simulink model "Pure_Pursuit_With_VFH"  (R2017b)
settings: Solver=FixedStepAuto  StartTime=0.0  StopTime=10.0  FixedStep=0.05  RelTol=1e-3
model workspace (MAT data in the model file):
  SL_ROS_VariableLengthArrays_MaxSizes.CommonInfo.ArrayTruncateAction = 'EmitWarning'
  SL_ROS_VariableLengthArrays_MaxSizes.MsgTypeMap = containers.Map
  SL_ROS_VariableLengthArrays_MaxSizes.MsgTypeMap.serialization.keys = {'sensor_msgs/LaserScan', 'std_msgs/Header'}
  SL_ROS_VariableLengthArrays_MaxSizes.MsgTypeMap.serialization.values{1}(1).PropertyName = 'Intensities'
  SL_ROS_VariableLengthArrays_MaxSizes.MsgTypeMap.serialization.values{1}(1).DataType = 'single'
  SL_ROS_VariableLengthArrays_MaxSizes.MsgTypeMap.serialization.values{1}(1).MaxLength = 721
  SL_ROS_VariableLengthArrays_MaxSizes.MsgTypeMap.serialization.values{1}(2).PropertyName = 'Ranges'
  SL_ROS_VariableLengthArrays_MaxSizes.MsgTypeMap.serialization.values{1}(2).DataType = 'single'
  SL_ROS_VariableLengthArrays_MaxSizes.MsgTypeMap.serialization.values{1}(2).MaxLength = 721
  SL_ROS_VariableLengthArrays_MaxSizes.MsgTypeMap.serialization.values{2}.PropertyName = 'FrameId'
  SL_ROS_VariableLengthArrays_MaxSizes.MsgTypeMap.serialization.values{2}.DataType = 'uint8'
  SL_ROS_VariableLengthArrays_MaxSizes.MsgTypeMap.serialization.values{2}.MaxLength = 720
  SL_ROS_VariableLengthArrays_MaxSizes.MsgTypeMap.serialization.uniformity = 0
  SL_ROS_VariableLengthArrays_MaxSizes.MsgTypeMap.serialization.keyType = 'char'
  SL_ROS_VariableLengthArrays_MaxSizes.MsgTypeMap.serialization.valueType = 'any'
  lookahead_dist = Simulink.Parameter
  lookahead_dist.Value = 2
  lookahead_dist.DataType = 'auto'
  lookahead_dist.Dimensions = [1 1]
undefined symbols (not defined in the file): Angular, Linear
libraries: robotlib x7, simulink x5, robotalgslib x2, simulink_extras x1, dspsigops x1
settings Model: ExplicitPartitioning=on  Creator=andrej  LastModifiedBy=andrej
settings OptimizationCC: PassReuseOutputArgsThreshold=0  MaxStackSize=64
settings DebuggingCC: ParameterTunabilityLossMsg=error
settings HardwareCC: ProdBitPerLong=64  ProdHWDeviceType=Intel->x86-64 (Linux 64)  UseEmbeddedCoderFeatures=off
settings SFSimCC: MATLABDynamicMemAlloc=off
settings RTWCC: SystemTargetFile=ert.tlc  HardwareBoard=Robot Operating System (ROS)  TemplateMakefile=ert_default_tmf  GenerateReport=on  Toolchain=Catkin  BuildConfiguration=Faster Runs  LaunchReport=on  TargetLang=C++
settings RTWCC: CustomInitializer=|
  | ros::NodeHandle private_nh = ros::NodeHandle("~");
  | 	ROS_INFO_STREAM("Node's namespace: " << private_nh.getNamespace());
  | 
  | // Tunable parameters of the Pure Pursuit algorithm
  | 	double desired_lin_vel;
  | 	if (private_nh.getParam("pure_pursuit/desired_lin_vel", desired_lin_vel))
  | 		this->Pure_Pursuit_With_VFH_P.PurePursuit_DesiredLinearVeloci = desired_lin_vel;
  | 	ROS_WARN_STREAM("Pure pursuit desired linear velocity set to " << this->Pure_Pursuit_With_VFH_P.PurePursuit_DesiredLinearVeloci << " m/s.");
  | 	double max_ang_vel;
  | 	if (private_nh.getParam("pure_pursuit/max_ang_vel", max_ang_vel))
  | 		this->Pure_Pursuit_With_VFH_P.PurePursuit_MaxAngularVelocity = max_ang_vel;
  | 	this->Pure_Pursuit_With_VFH_P.MaxAngularVelocity_Value = this->Pure_Pursuit_With_VFH_P.PurePursuit_MaxAngularVelocity;
  | 	double lookahead_dist;
  | 	if (private_nh.getParam("pure_pursuit/lookahead_dist", lookahead_dist))
  | 		this->Pure_Pursuit_With_VFH_P.PurePursuit_LookaheadDistance = lookahead_dist;
  | 
  | // Goal reach tolerance
  | 	double goal_radius;
  | 	if (private_nh.getParam("goal_radius", goal_radius))
  | 		this->Pure_Pursuit_With_VFH_P.GoalRadius_Value = goal_radius;
  | 
  | 
  | // Tunable parameters of the VFH algorithm
  | 
  | 	std::vector<double> range_dist;
  | 	if (private_nh.getParam("vfh/range_dist", range_dist)) {
  | 		this->Pure_Pursuit_With_VFH_P.VectorFieldHistogram_DistanceLi[0] = range_dist[0];
  | 		this->Pure_Pursuit_With_VFH_P.VectorFieldHistogram_DistanceLi[1] = range_dist[1];
  | 	}
  | 	std::vector<double> hist_thr;
  | 	if (private_nh.getParam("vfh/hist_thr", hist_thr)) {
  | 		this->Pure_Pursuit_With_VFH_P.VectorFieldHistogram_HistogramT[0] = hist_thr[0];
  | 		this->Pure_Pursuit_With_VFH_P.VectorFieldHistogram_HistogramT[1] = hist_thr[1];
  | 	}
  | 	double robot_radius;
  | 	if (private_nh.getParam("vfh/robot_radius", robot_radius))
  | 		this->Pure_Pursuit_With_VFH_P.VectorFieldHistogram_RobotRadiu = robot_radius;
  | 	double safety_dist;
  | 	if (private_nh.getParam("vfh/safety_dist", safety_dist))
  | 		this->Pure_Pursuit_With_VFH_P.VectorFieldHistogram_SafetyDist = safety_dist;
  | 	double min_turning_radius;
  | 	if (private_nh.getParam("vfh/min_turning_radius", min_turning_radius))
  | 		this->Pure_Pursuit_With_VFH_P.VectorFieldHistogram_MinTurning = min_turning_radius;
  | 	double target_dir_w;
  | 	if (private_nh.getParam("vfh/target_dir_w", target_dir_w))
  | 		this->Pure_Pursuit_With_VFH_P.VectorFieldHistogram_TargetDire = target_dir_w;
  | 	double current_dir_w;
  | 	if (private_nh.getParam("vfh/current_dir_w", current_dir_w))
  | 		this->Pure_Pursuit_With_VFH_P.VectorFieldHistogram_CurrentDir = current_dir_w;
  | 	double prev_dir_w;
  | 	if (private_nh.getParam("vfh/prev_dir_w", prev_dir_w))
  | 		this->Pure_Pursuit_With_VFH_P.VectorFieldHistogram_PreviousDi = prev_dir_w;
  | 
  | // Tunable parameters of the Linear Velocity Control
  | double double_param;
  | bool bool_param;
  | 
  | 	if (private_nh.getParam("velocity_profile/a", double_param))
  | 		this->Pure_Pursuit_With_VFH_P.LinVelocityControl_a = double_param;
  | 
  | 	if (private_nh.getParam("velocity_profile/c", double_param))
  | 		this->Pure_Pursuit_With_VFH_P.LinVelocityControl_c = double_param;
  | 
  |         if (private_nh.getParam("velocity_profile/k", double_param))
  | 		this->Pure_Pursuit_With_VFH_P.LinVelocityControl_k = double_param;
  | 
  | 	this->Pure_Pursuit_With_VFH_P.LinVelocityControl_omega_max = this->Pure_Pursuit_With_VFH_P.PurePursuit_MaxAngularVelocity;
  | 
  | 	if (private_nh.getParam("velocity_profile/v_max", double_param))
  | 		this->Pure_Pursuit_With_VFH_P.LinVelocityControl_v_max = double_param;
  | 
  | 	if (private_nh.getParam("velocity_profile/v_min", double_param))
  | 		this->Pure_Pursuit_With_VFH_P.LinVelocityControl_v_min = double_param;
  | 
  | 	if (private_nh.getParam("velocity_profile/enable", bool_param))
  | 		this->Pure_Pursuit_With_VFH_P.LinVelocityControl_enable = bool_param;
settings CodeAppCC: ForceParamTrailComments=on  OperatorAnnotations=on  StateflowObjectComments=on
settings ERTTargetCC: CodeReplacementLibrary=Intel IPP for x86-64 (Linux)  ERTCustomFileBanners=off  MultiInstanceERTCode=on  CodeInterfacePackaging=C++ class  SupportContinuousTime=on  SupportNonInlinedSFcns=on  RemoveResetFunc=off  ModelStepFunctionPrototypeControlCompliant=off  IndentSize=4

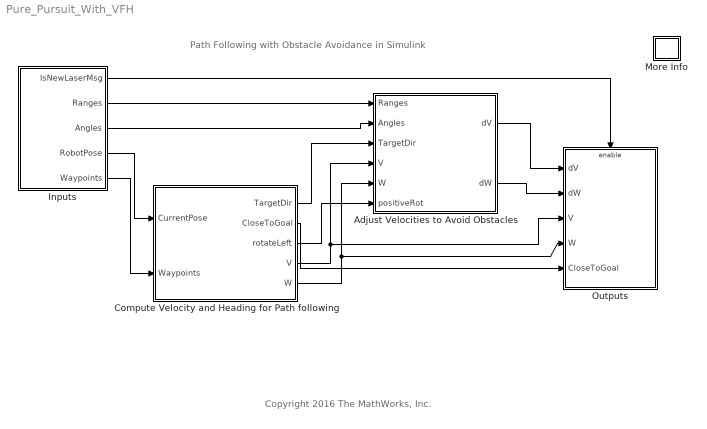
== system Pure_Pursuit_With_VFH ==
  note: Copyright 2016 The MathWorks, Inc.
  note: Path Following with Obstacle Avoidance in Simulink
  Adjust Velocities to Avoid Obstacles : Subsystem
  Compute Velocity and Heading for Path following : Subsystem
  Inputs : Subsystem
  More Info : Subsystem
      settings: OpenFcn=showdemo(bdroot(gcb))
      mask Display: disp('?')
  Outputs : Subsystem
  wires:
  Compute Velocity and Heading for Path following/2(CloseToGoal) -> Outputs/5(CloseToGoal)
  Inputs/5(Waypoints) -> Compute Velocity and Heading for Path following/2(Waypoints)
  Inputs/4(RobotPose) -> Compute Velocity and Heading for Path following/1(CurrentPose)
  Inputs/1(IsNewLaserMsg) -> Outputs/Enable
  Inputs/2(Ranges) -> Adjust Velocities to Avoid Obstacles/1(Ranges)
  Adjust Velocities to Avoid Obstacles/2(dW) -> Outputs/2(dW)
  Compute Velocity and Heading for Path following/1(TargetDir) -> Adjust Velocities to Avoid Obstacles/3(TargetDir)
  Inputs/3(Angles) -> Adjust Velocities to Avoid Obstacles/2(Angles)
  Compute Velocity and Heading for Path following/3(rotateLeft) -> Adjust Velocities to Avoid Obstacles/6(positiveRot)
  Adjust Velocities to Avoid Obstacles/1(dV) -> Outputs/1(dV)
  Compute Velocity and Heading for Path following/5(W) -> Adjust Velocities to Avoid Obstacles/5(W), Outputs/4(W)
  Compute Velocity and Heading for Path following/4(V) -> Adjust Velocities to Avoid Obstacles/4(V), Outputs/3(V)

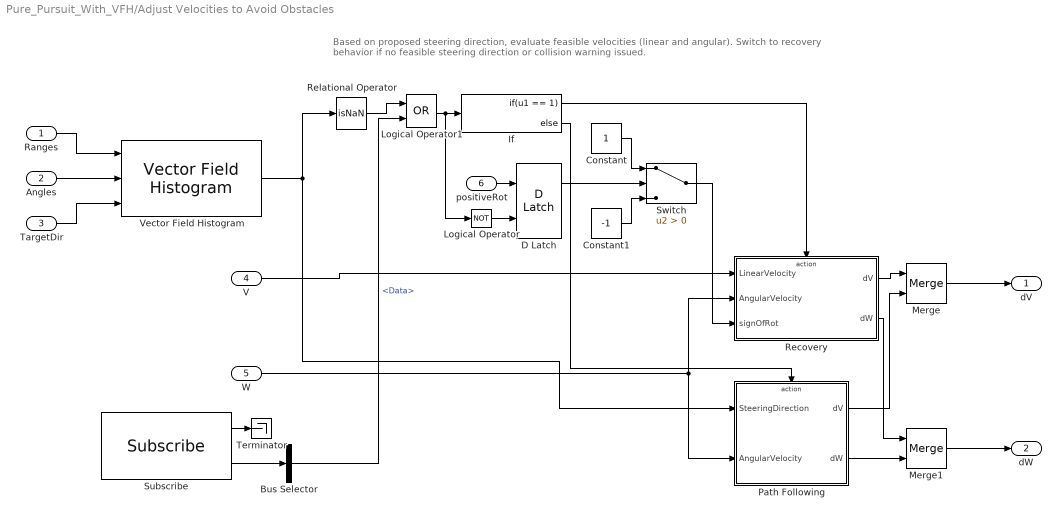
== system Pure_Pursuit_With_VFH/Adjust Velocities to Avoid Obstacles ==
  note: Based on proposed steering direction, evaluate feasible velocities (linear and angular).
      | 	Switch to recovery behavior if no feasible steering direction or collision warning issued.
  Ranges : Inport
  Angles : Inport  Port=2
  TargetDir : Inport  Port=3
  V : Inport  Port=4
  W : Inport  Port=5
  positiveRot : Inport  Port=6
  Bus Selector : BusSelector  OutputSignals=Data
  Constant : Constant
  Constant1 : Constant  Value=-1
  D Latch : simulink_extras/Flip Flops/D Latch
      settings: SourceProductName=Simulink  SourceProductBaseCode=SL
  If : If  IfExpression=u1 == 1
  Logical Operator : Logic  Operator=NOT  IconShape=distinctive  AllPortsSameDT=off  OutDataTypeStr=boolean
  Logical Operator1 : Logic  Operator=OR  AllPortsSameDT=off  OutDataTypeStr=boolean
  Merge : Merge
  Merge1 : Merge
  Path Following : Subsystem  TreatAsAtomicUnit=on
  Recovery : Subsystem  TreatAsAtomicUnit=on
  Relational Operator : RelationalOperator  Operator=isNaN  OutDataTypeStr=boolean  RndMeth=Simplest
  Subscribe : robotlib/Subscribe  SourceLibraryInfo=This block requires Robotics System Toolbox  topicSource=Specify your own  topic=/Collision_warning  messageType=std_msgs/Bool  sampleTime=-1  messageQueueLength=1
      settings: SourceProductBaseCode=RO
  Switch : Switch  Criteria=u2 > Threshold
  Terminator : Terminator
  Vector Field Histogram : robotalgslib/Vector Field Histogram  NumAngularSectors=240  DistanceLimits=[ 0.05, 2.0 ]  HistogramThresholds=[ 3, 6 ]  RobotRadius=0.3  SafetyDistance=0.1  MinTurningRadius=0.3  SimulateUsing=Code generation  TargetDirectionWeight=5  CurrentDirectionWeight=2  PreviousDirectionWeight=2
      settings: SourceProductName=Robotics System Toolbox  SourceProductBaseCode=RO
  dV : Outport
  dW : Outport  Port=2
  wires:
  Merge1/1 -> dW/1
  V/1 -> Recovery/1(LinearVelocity)
  Vector Field Histogram/1 -> Path Following/1(SteeringDirection), Relational Operator/1
  W/1 -> Path Following/2(AngularVelocity), Recovery/2(AngularVelocity)
  Angles/1 -> Vector Field Histogram/2
  Merge/1 -> dV/1
  TargetDir/1 -> Vector Field Histogram/3
  Ranges/1 -> Vector Field Histogram/1
  If/1 -> Recovery/Action
  If/2 -> Path Following/Action
  Recovery/2(dW) -> Merge1/1
  Path Following/2(dW) -> Merge1/2
  Recovery/1(dV) -> Merge/1
  Path Following/1(dV) -> Merge/2
  Subscribe/2 -> Bus Selector/1
  Subscribe/1 -> Terminator/1
  Logical Operator1/1 -> Logical Operator/1, If/1
  Relational Operator/1 -> Logical Operator1/1
  Bus Selector/1 -> Logical Operator1/2  "<Data>"
  Logical Operator/1 -> D Latch/2
  positiveRot/1 -> D Latch/1
  D Latch/1 -> Switch/2
  Switch/1 -> Recovery/3(signOfRot)
  Constant/1 -> Switch/1
  Constant1/1 -> Switch/3

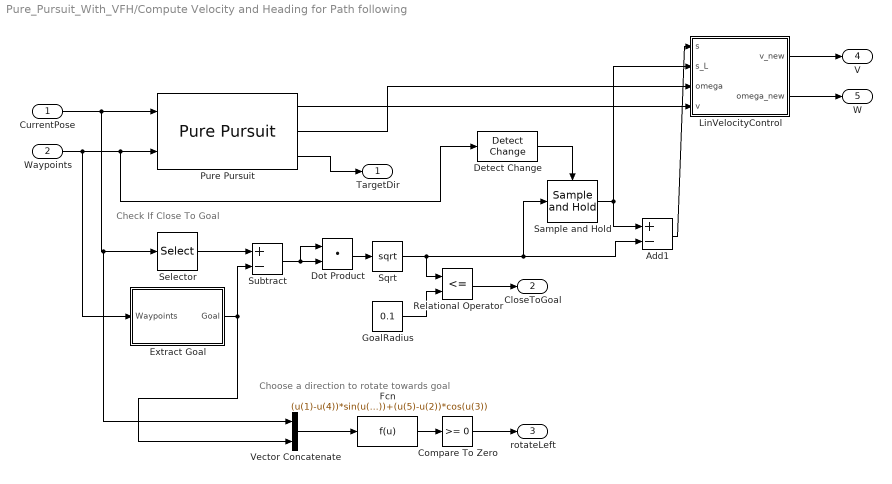
== system Pure_Pursuit_With_VFH/Compute Velocity and Heading for Path following ==
  note: Choose a direction to rotate towards goal
  note: Check If Close To Goal
  CurrentPose : Inport
  Waypoints : Inport  Port=2
  " Extract Goal" : MATLAB Function  TreatAsAtomicUnit=on
  Add1 : Sum  Inputs=+-
  Compare To Zero : simulink/Logic and Bit Operations/Compare To Zero  relop=>=  OutDataTypeStr=boolean
  Detect Change : simulink/Logic and Bit Operations/Detect Change  vinit=true  OutDataTypeStr=boolean
  Dot Product : DotProduct  InputSameDT=on  OutDataTypeStr=Inherit: Inherit via internal rule
  Fcn : Fcn  Expr=(u(1)-u(4))*sin(u(3))+(u(5)-u(2))*cos(u(3))
  GoalRadius : Constant  Value=0.1
  LinVelocityControl : Subsystem  mask(Desired velocity profile){v_min=0.2, v_max=0.9, omega_max=1.0, c=0.5, a=0.3, k=10, enable=on}
      mask prompts: v_min "v_min [m/s]"; v_max "v_max [m/s]"; omega_max "omega_max [rad/s]"; c "c [m]"; a "a [m/s^2]"; k "Prefilter constant k"; enable "enable control"
      mask help:
      | Robot moves with velocity v_min around the waypoints (+/- c) and accelerating with constant acceleration (a) in between.
      | Maximum speed is  v_max.
      | Reference prefilter has the transfer function of the form k/(s+k).
      | Enable control to change velocity according to this profile, otherwise pass through velocity inputs.
  Pure Pursuit : robotalgslib/Pure Pursuit  DesiredLinearVelocity=0.3  MaxAngularVelocity=1.0  LookaheadDistance=1.0  TargetDirPort=on  SimulateUsing=Code generation
      settings: SourceProductName=Robotics System Toolbox  SourceProductBaseCode=RO
  Relational Operator : RelationalOperator  Operator=<=  OutDataTypeStr=boolean  RndMeth=Simplest
  Sample and Hold : dspsigops/Sample and Hold  trig=Rising edge  initCond=0  latchinput=off
  Selector : Selector  InputPortWidth=3  IndexOptions=Index vector (dialog)  Indices=[1 2]  OutputSizes=1
  Sqrt : Sqrt  SaturateOnIntegerOverflow=on
  Subtract : Sum  Inputs=+-
  Vector Concatenate : Concatenate
  TargetDir : Outport
  CloseToGoal : Outport  Port=2
  rotateLeft : Outport  Port=3
  V : Outport  Port=4
  W : Outport  Port=5
  wires:
  Pure Pursuit/3 -> TargetDir/1
  Waypoints/1 -> " Extract Goal"/1(Waypoints), Detect Change/1, Pure Pursuit/2
  CurrentPose/1 -> Vector Concatenate/1, Selector/1, Pure Pursuit/1
  Relational Operator/1 -> CloseToGoal/1
  GoalRadius/1 -> Relational Operator/2
  Selector/1 -> Subtract/1
  Dot Product/1 -> Sqrt/1
  Sqrt/1 -> Sample and Hold/1, Add1/2, Relational Operator/1
  Subtract/1 -> Dot Product/1, Dot Product/2
  " Extract Goal"/1(Goal) -> Subtract/2, Vector Concatenate/2
  Vector Concatenate/1 -> Fcn/1
  Fcn/1 -> Compare To Zero/1
  Compare To Zero/1 -> rotateLeft/1
  Detect Change/1 -> Sample and Hold/Trigger
  Sample and Hold/1 -> Add1/1, LinVelocityControl/2(s_L)
  Add1/1 -> LinVelocityControl/1(s)
  LinVelocityControl/1(v_new) -> V/1
  LinVelocityControl/2(omega_new) -> W/1
  Pure Pursuit/2 -> LinVelocityControl/3(omega)
  Pure Pursuit/1 -> LinVelocityControl/4(v)

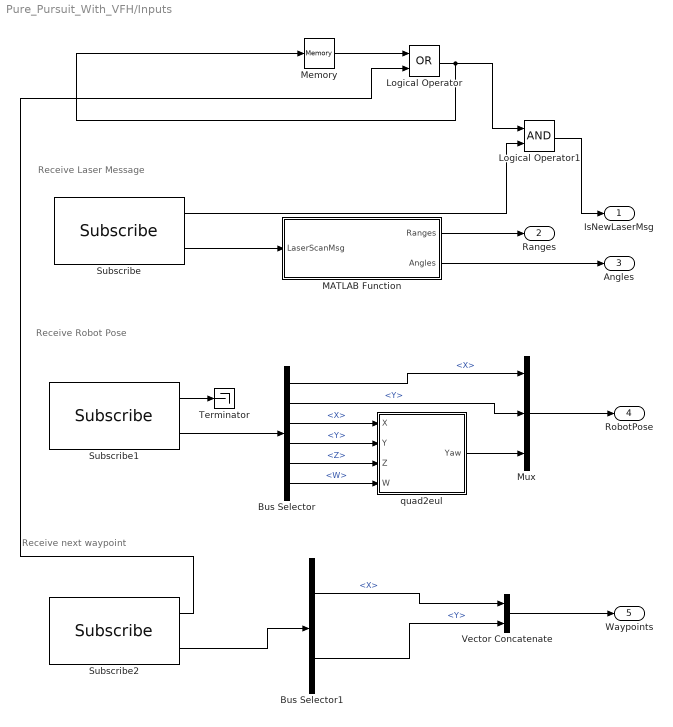
== system Pure_Pursuit_With_VFH/Inputs ==
  note: Receive next waypoint
  note: Receive Robot Pose
  note: Receive Laser Message
  Bus Selector : BusSelector  OutputSignals=Pose.Pose.Position.X,Pose.Pose.Position.Y,Pose.Pose.Orientation.X,Pose.Pose.Orientation.Y,Pose.Pose.Orientation.Z,Pose.Pose.Orientation.W
  Bus Selector1 : BusSelector  OutputSignals=X,Y
  Logical Operator : Logic  Operator=OR  AllPortsSameDT=off  OutDataTypeStr=boolean
  Logical Operator1 : Logic  AllPortsSameDT=off  OutDataTypeStr=boolean
  MATLAB Function : MATLAB Function  TreatAsAtomicUnit=on
  Memory : Memory
  Mux : Mux  Inputs=3
  Subscribe : robotlib/Subscribe  SourceLibraryInfo=This block requires Robotics System Toolbox  topicSource=Select from ROS network  topic=/scan  messageType=sensor_msgs/LaserScan  sampleTime=-1  messageQueueLength=1
      settings: SourceProductBaseCode=RO
  Subscribe1 : robotlib/Subscribe  SourceLibraryInfo=This block requires Robotics System Toolbox  topicSource=Specify your own  topic=/current_pose  messageType=nav_msgs/Odometry  sampleTime=-1  messageQueueLength=1
      settings: SourceProductBaseCode=RO
  Subscribe2 : robotlib/Subscribe  SourceLibraryInfo=This block requires Robotics System Toolbox  topicSource=Specify your own  topic=/next_waypoint  messageType=geometry_msgs/Point  sampleTime=-1  messageQueueLength=1
      settings: SourceProductBaseCode=RO
  Terminator : Terminator
  Vector Concatenate : Concatenate  Mode=Multidimensional array  ConcatenateDimension=2
  quad2eul : MATLAB Function  TreatAsAtomicUnit=on
  IsNewLaserMsg : Outport
  Ranges : Outport  Port=2
  Angles : Outport  Port=3
  RobotPose : Outport  Port=4
  Waypoints : Outport  Port=5
  wires:
  Subscribe/2 -> MATLAB Function/1(LaserScanMsg)
  quad2eul/1(Yaw) -> Mux/3
  Subscribe1/2 -> Bus Selector/1
  Bus Selector/3 -> quad2eul/1(X)  "<X>"
  Subscribe1/1 -> Terminator/1
  Bus Selector/2 -> Mux/2  "<Y>"
  Bus Selector/5 -> quad2eul/3(Z)  "<Z>"
  Bus Selector/4 -> quad2eul/2(Y)  "<Y>"
  Bus Selector/1 -> Mux/1  "<X>"
  Bus Selector/6 -> quad2eul/4(W)  "<W>"
  MATLAB Function/1(Ranges) -> Ranges/1
  MATLAB Function/2(Angles) -> Angles/1
  Subscribe/1 -> Logical Operator1/2
  Mux/1 -> RobotPose/1
  Subscribe2/2 -> Bus Selector1/1
  Bus Selector1/1 -> Vector Concatenate/1  "<X>"
  Bus Selector1/2 -> Vector Concatenate/2  "<Y>"
  Vector Concatenate/1 -> Waypoints/1
  Memory/1 -> Logical Operator/1
  Logical Operator/1 -> Logical Operator1/1, Memory/1
  Subscribe2/1 -> Logical Operator/2
  Logical Operator1/1 -> IsNewLaserMsg/1

== system Pure_Pursuit_With_VFH/More Info ==

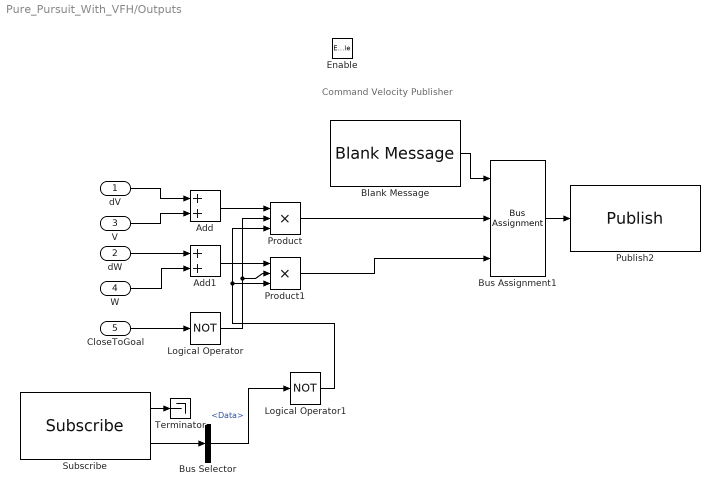
== system Pure_Pursuit_With_VFH/Outputs ==
  note: Command Velocity Publisher
  dV : Inport
  dW : Inport  Port=2
  V : Inport  Port=3
  W : Inport  Port=4
  CloseToGoal : Inport  Port=5
  Enable : EnablePort
  Add : Sum
  Add1 : Sum
  Blank Message : robotlib/Blank Message  SourceLibraryInfo=This block requires Robotics System Toolbox  messageType=geometry_msgs/Twist  SampleTime=inf
      settings: SourceProductBaseCode=RO
  Bus Assignment1 : BusAssignment  DialogController=Simulink.DDGSource_BusAssignment  AssignedSignals=Linear.X,Angular.Z
  Bus Selector : BusSelector  OutputSignals=Data
  Logical Operator : Logic  Operator=NOT  AllPortsSameDT=off  OutDataTypeStr=boolean
  Logical Operator1 : Logic  Operator=NOT  AllPortsSameDT=off  OutDataTypeStr=boolean
  Product : Product  Inputs=3
  Product1 : Product  Inputs=3
  Publish2 : robotlib/Publish  SourceLibraryInfo=This block requires Robotics System Toolbox  topicSource=Select from ROS network  topic=/mobile_base/commands/velocity  messageType=geometry_msgs/Twist  messageQueueLength=1
      settings: SourceProductBaseCode=RO
  Subscribe : robotlib/Subscribe  SourceLibraryInfo=This block requires Robotics System Toolbox  topicSource=Specify your own  topic=/emergency_stop  messageType=std_msgs/Bool  sampleTime=-1  messageQueueLength=1
      settings: SourceProductBaseCode=RO
  Terminator : Terminator
  wires:
  V/1 -> Add/2
  W/1 -> Add1/2
  dV/1 -> Add/1
  dW/1 -> Add1/1
  CloseToGoal/1 -> Logical Operator/1
  Add/1 -> Product/1
  Add1/1 -> Product1/1
  Product1/1 -> Bus Assignment1/3
  Product/1 -> Bus Assignment1/2
  Blank Message/1 -> Bus Assignment1/1
  Bus Assignment1/1 -> Publish2/1
  Logical Operator/1 -> Product1/2, Product/2
  Logical Operator1/1 -> Product1/3, Product/3
  Subscribe/2 -> Bus Selector/1
  Bus Selector/1 -> Logical Operator1/1  "<Data>"
  Subscribe/1 -> Terminator/1

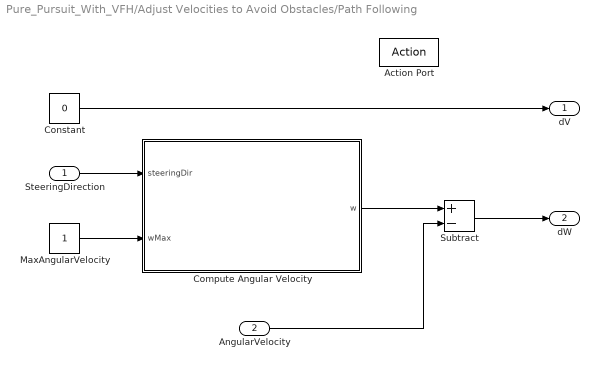
== system Pure_Pursuit_With_VFH/Adjust Velocities to Avoid Obstacles/Path Following ==
  SteeringDirection : Inport
  AngularVelocity : Inport  Port=2
  Action Port : ActionPort  ActionType=else
  Compute Angular Velocity : MATLAB Function  TreatAsAtomicUnit=on
  Constant : Constant  Value=0
  MaxAngularVelocity : Constant
  Subtract : Sum  Inputs=+-
  dV : Outport
  dW : Outport  Port=2
  wires:
  Constant/1 -> dV/1
  MaxAngularVelocity/1 -> Compute Angular Velocity/2(wMax)
  SteeringDirection/1 -> Compute Angular Velocity/1(steeringDir)
  Subtract/1 -> dW/1
  Compute Angular Velocity/1(w) -> Subtract/1
  AngularVelocity/1 -> Subtract/2

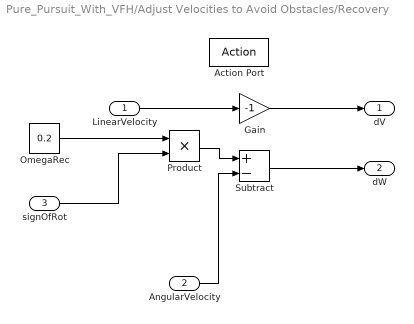
== system Pure_Pursuit_With_VFH/Adjust Velocities to Avoid Obstacles/Recovery ==
  LinearVelocity : Inport
  AngularVelocity : Inport  Port=2
  signOfRot : Inport  Port=3
  Action Port : ActionPort  ActionType=then
  Gain : Gain  Gain=-1
  OmegaRec : Constant  Value=0.2
  Product : Product
  Subtract : Sum  Inputs=+-
  dV : Outport
  dW : Outport  Port=2
  wires:
  LinearVelocity/1 -> Gain/1
  Gain/1 -> dV/1
  Subtract/1 -> dW/1
  OmegaRec/1 -> Product/1
  Product/1 -> Subtract/1
  AngularVelocity/1 -> Subtract/2
  signOfRot/1 -> Product/2

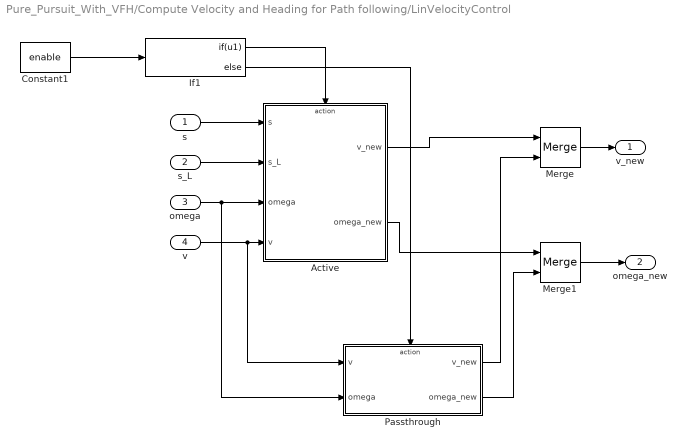
== system Pure_Pursuit_With_VFH/Compute Velocity and Heading for Path following/LinVelocityControl ==
  s : Inport
  s_L : Inport  Port=2
  omega : Inport  Port=3
  v : Inport  Port=4
  Active : Subsystem  TreatAsAtomicUnit=on
      mask Display: image('Vel_Profile.svg');
  Constant1 : Constant  Value=enable  OutDataTypeStr=boolean
  If1 : If  IfExpression=u1
  Merge : Merge
  Merge1 : Merge
  Passthrough : Subsystem  TreatAsAtomicUnit=on
  v_new : Outport
  omega_new : Outport  Port=2
  wires:
  s/1 -> Active/1(s)
  s_L/1 -> Active/2(s_L)
  omega/1 -> Passthrough/2(omega), Active/3(omega)
  v/1 -> Passthrough/1(v), Active/4(v)
  Constant1/1 -> If1/1
  If1/1 -> Active/Action
  If1/2 -> Passthrough/Action
  Merge/1 -> v_new/1
  Active/1(v_new) -> Merge/1
  Passthrough/1(v_new) -> Merge/2
  Active/2(omega_new) -> Merge1/1
  Passthrough/2(omega_new) -> Merge1/2
  Merge1/1 -> omega_new/1

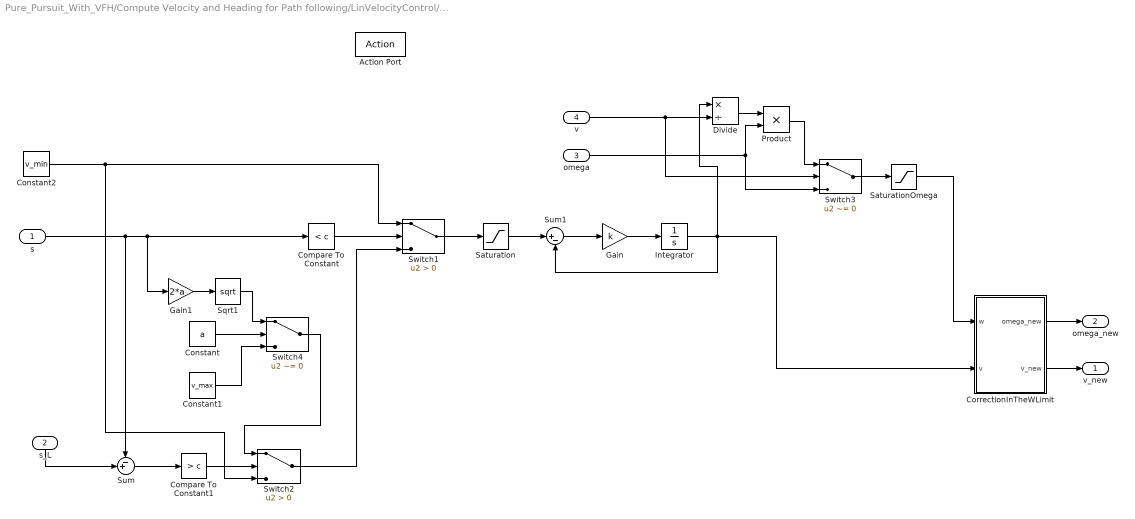
== system Pure_Pursuit_With_VFH/Compute Velocity and Heading for Path following/LinVelocityControl/Active ==
  s : Inport
  s_L : Inport  Port=2
  omega : Inport  Port=3
  v : Inport  Port=4
  Action Port : ActionPort  ActionType=then
  Compare To Constant : simulink/Logic and Bit Operations/Compare To Constant  relop=<  const=c  OutDataTypeStr=boolean
  Compare To Constant1 : simulink/Logic and Bit Operations/Compare To Constant  relop=>  const=c  OutDataTypeStr=boolean
  Constant : Constant  Value=a
  Constant1 : Constant  Value=v_max
  Constant2 : Constant  Value=v_min
  CorrectionInTheWLimit : Subsystem
  Divide : Product  Inputs=*/
  Gain : Gain  Gain=k
  Gain1 : Gain  Gain=2*a
  Integrator : Integrator
  Product : Product
  Saturation : Saturate  UpperLimit=v_max  LowerLimit=-v_max
  SaturationOmega : Saturate  UpperLimit=omega_max  LowerLimit=-omega_max
  Sqrt1 : Sqrt  SaturateOnIntegerOverflow=on
  Sum : Sum  Inputs=-+|
  Sum1 : Sum  Inputs=|+-
  Switch1 : Switch  Criteria=u2 > Threshold
  Switch2 : Switch  Criteria=u2 > Threshold
  Switch3 : Switch  Criteria=u2 ~= 0
  Switch4 : Switch  Criteria=u2 ~= 0
  v_new : Outport
  omega_new : Outport  Port=2
  wires:
  Divide/1 -> Product/1
  Switch1/1 -> Saturation/1
  Compare To Constant1/1 -> Switch2/2
  omega/1 -> Switch3/3, Product/2
  v/1 -> Divide/2, Switch3/2
  Compare To Constant/1 -> Switch1/2
  s_L/1 -> Sum/2
  Constant2/1 -> Switch1/1, Switch2/3
  Product/1 -> Switch3/1
  Sum/1 -> Compare To Constant1/1
  Saturation/1 -> Sum1/1
  Switch2/1 -> Switch1/3
  Switch3/1 -> SaturationOmega/1
  SaturationOmega/1 -> CorrectionInTheWLimit/1(w)
  Constant1/1 -> Switch4/3
  Sqrt1/1 -> Switch4/1
  Gain1/1 -> Sqrt1/1
  Constant/1 -> Switch4/2
  s/1 -> Gain1/1, Compare To Constant/1, Sum/1
  Switch4/1 -> Switch2/1
  Gain/1 -> Integrator/1
  Sum1/1 -> Gain/1
  Integrator/1 -> CorrectionInTheWLimit/2(v), Divide/1, Sum1/2
  CorrectionInTheWLimit/1(omega_new) -> omega_new/1
  CorrectionInTheWLimit/2(v_new) -> v_new/1

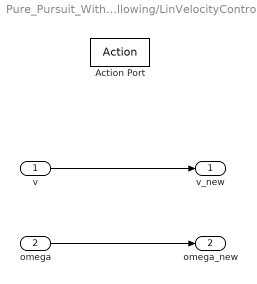
== system Pure_Pursuit_With_VFH/Compute Velocity and Heading for Path following/LinVelocityControl/Passthrough ==
  v : Inport
  omega : Inport  Port=2
  Action Port : ActionPort  ActionType=else
  v_new : Outport
  omega_new : Outport  Port=2
  wires:
  omega/1 -> omega_new/1
  v/1 -> v_new/1

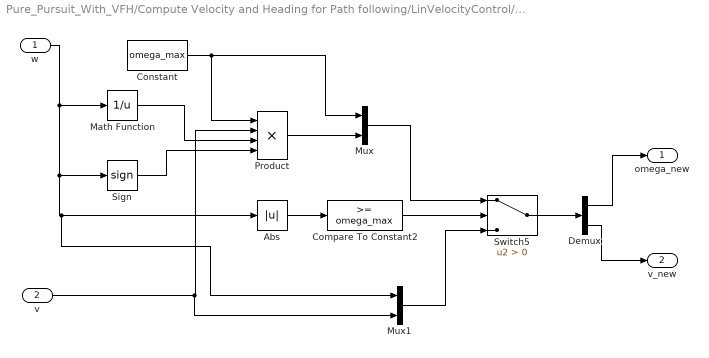
== system Pure_Pursuit_With_VFH/Compute Velocity and Heading for Path following/LinVelocityControl/Active/CorrectionInTheWLimit ==
  w : Inport
  v : Inport  Port=2
  Abs : Abs
  Compare To Constant2 : simulink/Logic and Bit Operations/Compare To Constant  relop=>=  const=omega_max  OutDataTypeStr=boolean
  Constant : Constant  Value=omega_max
  Demux : Demux  Outputs=2
  Math Function : Math  Operator=reciprocal  SaturateOnIntegerOverflow=on
  Mux : Mux  Inputs=2
  Mux1 : Mux  Inputs=2
  Product : Product  Inputs=4
  Sign : Signum
  Switch5 : Switch  Criteria=u2 > Threshold
  omega_new : Outport
  v_new : Outport  Port=2
  wires:
  w/1 -> Mux1/1, Abs/1, Sign/1, Math Function/1
  Compare To Constant2/1 -> Switch5/2
  Abs/1 -> Compare To Constant2/1
  Mux/1 -> Switch5/1
  Constant/1 -> Product/1, Mux/1
  v/1 -> Mux1/2, Product/2
  Math Function/1 -> Product/3
  Product/1 -> Mux/2
  Mux1/1 -> Switch5/3
  Switch5/1 -> Demux/1
  Demux/1 -> omega_new/1
  Demux/2 -> v_new/1
  Sign/1 -> Product/4

== matlab function Pure_Pursuit_With_VFH/Inputs/quad2eul ==
  data: X input; Yaw output; Y input; Z input; W input
function Yaw = quat2eulBlk(X, Y, Z, W)
%#codegen

eularAngles = quat2eul([W, X, Y, Z]);
Yaw = eularAngles(1);

== matlab function Pure_Pursuit_With_VFH/Inputs/MATLAB Function ==
  data: LaserScanMsg input; Ranges output; Angles output
function [Ranges, Angles] = ExtractRangeData(LaserScanMsg)
%#codegen

% Extract Range information
Ranges = double(LaserScanMsg.Ranges);

% Construct Angles vector using AngleMin and AngleIncrement from sensor
% reading.
angMin = double(LaserScanMsg.AngleMin);
angIncrement = double(LaserScanMsg.AngleIncrement);

numReadings = numel(Ranges);
rawAngles = angMin + (0:numReadings-1)' * angIncrement;

% Wrap the angles to the (-pi,pi] interval.
Angles = robotics.internal.wrapToPi(double(rawAngles));

== matlab function Pure_Pursuit_With_VFH/Compute Velocity and Heading for Path following/ Extract Goal ==
  data: Waypoints input; Goal output
function Goal = extractGoal(Waypoints)
%#codegen
%b = isnan(Waypoints);
%[rows,~] = find(b);
%ridx = setdiff(1:size(Waypoints,1), sort(rows));
%Goal = [Waypoints(ridx(end), 1) Waypoints(ridx(end), 2)];

% Goal = next waypoint (X, Y coordinate)
Goal = [Waypoints(end, 1) Waypoints(end, 2)];

== matlab function Pure_Pursuit_With_VFH/Adjust Velocities to Avoid Obstacles/Path Following/Compute Angular Velocity ==
  data: steeringDir input; w output; wMax input
function w = exampleHelperComputeAngularVelocity(steeringDir, wMax)
%EXAMPLEHELPERCOMPUTEANGULARVELOCITY Compute angular velocity
%   W = exampleHelperComputeAngularVelocity(STEERINGDIR)
%   returns the angular velocity W for a differential drive robot in radians
%   per second for a given steering direction STEERINGDIR in the robot's
%   coordinate frame in radians.
%
%   W = exampleHelperComputeAngularVelocity(STEERINGDIR, WMAX)
%   returns the angular velocity W for a differential drive robot in radians
%   per second for a given steering direction STEERINGDIR in the robot's
%   coordinate frame in radians and maximum angular velocity WMAX in
%   radians per second. The output angular velocity is saturated based on
%   the WMAX.
%
%   Example:
%       
%       w = exampleHelperComputeAngularVelocity(0.2, 1);

% Copyright 2015 The MathWorks, Inc.

%#codegen
%#ok<*EMCA>

% Allow variable input arguments
if nargin == 1   
    wMax = inf;
end

validateattributes(steeringDir, {'double'},{'real'},...
    'exampleHelperComputeAngularVelocity', 'STEERINGDIR', 1);
validateattributes(wMax, {'double'},{'real', 'positive'},...
    'exampleHelperComputeAngularVelocity', 'WMAX', 2);

% Computing in robot's coordinate frame
curPose = [0 0 0];

% The following computation is similar to robotics.PurePursuit
lookaheadPoint = [cos(steeringDir), sin(steeringDir)];
slope = atan2((lookaheadPoint(2) - curPose(2)), ...
    (lookaheadPoint(1) - curPose(1)));
alpha = angdiff(curPose(3), slope);

% Angular velocity command for a differential drive robot is
% equal to the desired curvature to be followed by the robot.

w = (2*sin(alpha));

% Pick a constant rotation when robot is facing in the opposite
% direction of the path
if abs(abs(alpha) - pi) < 1e-12
    w = sign(w)*1;
end

if abs(w) > wMax
    w = sign(w)*wMax;
end

end
